simulink model "Atividade"  (R2018b)
settings: Solver=VariableStepAuto  StartTime=0.0  StopTime=10  RelTol=1e-3
undefined symbols (not defined in the file): T
settings Model: Creator=18.01226-4  LastModifiedBy=18.01226-4

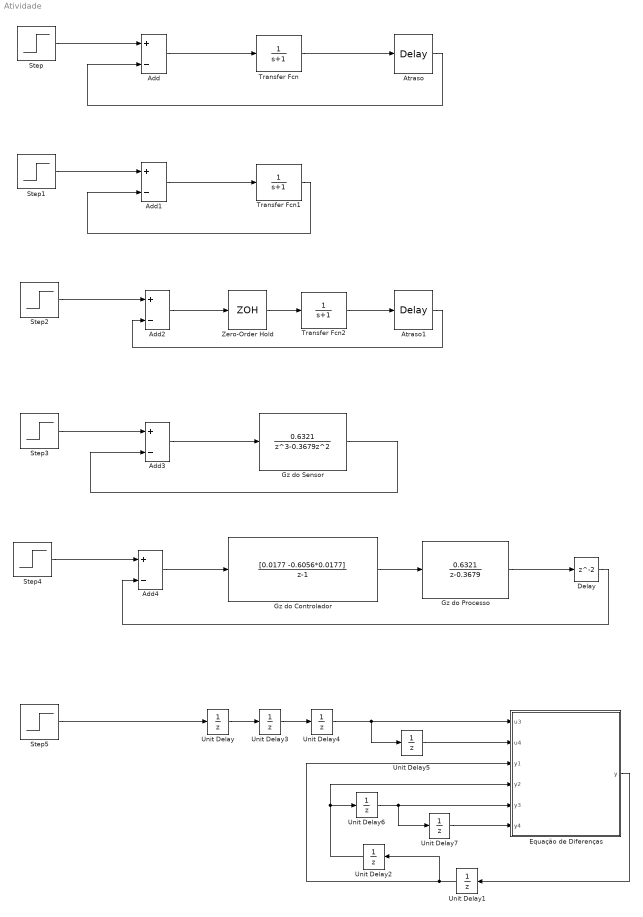
== system Atividade ==
  Add{,1..4} (5 alike) : Sum  Inputs=+-
  Atraso : TransportDelay  DelayTime=2
  Atraso1 : TransportDelay  DelayTime=2
  Delay : Delay
  Equação de Diferenças : MATLAB Function  TreatAsAtomicUnit=on
  Gz do Controlador : DiscreteTransferFcn  Numerator=[0.0177 -0.6056*0.0177]  Denominator=[1 -1]  SampleTime=T
  "Gz do Processo " : DiscreteTransferFcn  Numerator=[0.6321]  Denominator=[1 -0.3679]  SampleTime=T
  "Gz do Sensor " : DiscreteTransferFcn  Numerator=[0.6321]  Denominator=[1 -0.3679 0 0]  SampleTime=T
  Step{,1..5} (6 alike) : Step  SampleTime=0
  Transfer Fcn : TransferFcn  Denominator=[1 1]
  Transfer Fcn1 : TransferFcn  Denominator=[1 1]
  Transfer Fcn2 : TransferFcn  Denominator=[1 1]
  Unit Delay{,1..7} (8 alike) : UnitDelay  SampleTime=T
  Zero-Order Hold : ZeroOrderHold  SampleTime=-1
  wires:
  Step/1 -> Add/1
  Add/1 -> Transfer Fcn/1
  Transfer Fcn/1 -> Atraso/1
  Atraso/1 -> Add/2
  Transfer Fcn1/1 -> Add1/2
  Step1/1 -> Add1/1
  Add1/1 -> Transfer Fcn1/1
  Transfer Fcn2/1 -> Atraso1/1
  Step2/1 -> Add2/1
  Add2/1 -> Zero-Order Hold/1
  Zero-Order Hold/1 -> Transfer Fcn2/1
  Atraso1/1 -> Add2/2
  "Gz do Sensor "/1 -> Add3/2
  Step3/1 -> Add3/1
  Add3/1 -> "Gz do Sensor "/1
  Add4/1 -> Gz do Controlador/1
  "Gz do Processo "/1 -> Delay/1
  Step4/1 -> Add4/1
  Delay/1 -> Add4/2
  Gz do Controlador/1 -> "Gz do Processo "/1
  Step5/1 -> Unit Delay/1
  Equação de Diferenças/1(y) -> Unit Delay1/1
  Unit Delay1/1 -> Unit Delay2/1, Equação de Diferenças/3(y1)
  Unit Delay2/1 -> Unit Delay6/1, Equação de Diferenças/4(y2)
  Unit Delay/1 -> Unit Delay3/1
  Unit Delay3/1 -> Unit Delay4/1
  Unit Delay4/1 -> Unit Delay5/1, Equação de Diferenças/1(u3)
  Unit Delay5/1 -> Equação de Diferenças/2(u4)
  Unit Delay6/1 -> Unit Delay7/1, Equação de Diferenças/5(y3)
  Unit Delay7/1 -> Equação de Diferenças/6(y4)

== matlab function Atividade/Equação de Diferenças ==
  data: u3 input; y output; u4 input; y1 input; y2 input; y3 input; y4 input
function y = fcn(u3,u4,y1,y2,y3,y4)

y = 0.01119*u3 - 0.006776*u4 + 1.368*y1 - 0.3679*y2 - 0.01119*y3 + 0.006776*y4;
